simulink model "TTS2_EXT"  (R2024b)
settings: Solver=FixedStepAuto  StartTime=0.0  StopTime=inf  FixedStep=0.01  RelTol=1e-3
model workspace (MAT data in the model file):
  amp_f1 = -100
  amp_f10 = 0.5
  amp_f11 = -0.1
  amp_f12 = 1
  amp_f13 = 0.5
  amp_f14 = -20
  amp_f15 = 0.5
  amp_f16 = 0.5
  amp_f17 = 20
  amp_f18 = -30
  amp_f19 = 0.1
  amp_f2 = -20
  amp_f20 = -20
  amp_f21 = 20
  amp_f3 = -30
  amp_f4 = -30
  amp_f5 = -10
  amp_f51 = -10
  amp_f52 = -30
  amp_f53 = -30
  amp_f54 = 20
  amp_f55 = -100
  amp_f6 = -30
  amp_f7 = -30
  amp_f8 = -30
  amp_f9 = 1
  from_f1 = 570
  from_f10 = 5970
  from_f11 = 6570
  from_f12 = 7170
  from_f13 = 7770
  from_f14 = 8370
  from_f15 = 8970
  from_f16 = 9570
  from_f17 = 10170
  from_f18 = 10770
  from_f19 = 11370
  from_f2 = 1170
  from_f20 = 11970
  from_f21 = 12570
  from_f3 = 1770
  from_f4 = 2370
  from_f5 = 2970
  from_f51 = 13170
  from_f52 = 13770
  from_f53 = 14370
  from_f54 = 14970
  from_f55 = 15570
  from_f6 = 3570
  from_f7 = 4170
  from_f8 = 4770
  from_f9 = 5370
libraries: simulink x52, lab310_library x26, opclib x3
(part 1 of 3)
settings Model: Creator=tanas  LastModifiedBy=pchoi
settings DataIOCC: ReturnWorkspaceOutputs=off
settings OptimizationCC: ReuseModelBlockBuffer=off
settings DebuggingCC: UnconnectedInputMsg=warning  UnconnectedOutputMsg=warning  UnconnectedLineMsg=warning  ArithmeticOperatorsInVariantConditions=warning
settings ModelReferenceCC: EnableRefExpFcnMdlSchedulingChecks=on
settings SFSimCC: CustomCodeUndefinedFunction=UseInterfaceOnly
settings RTWCC: GPUComputeCapability=3.5

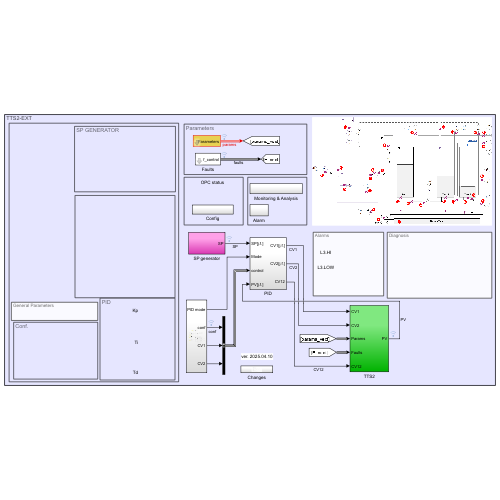
[thumbnail: Simulink's stored preview of the top-level diagram]
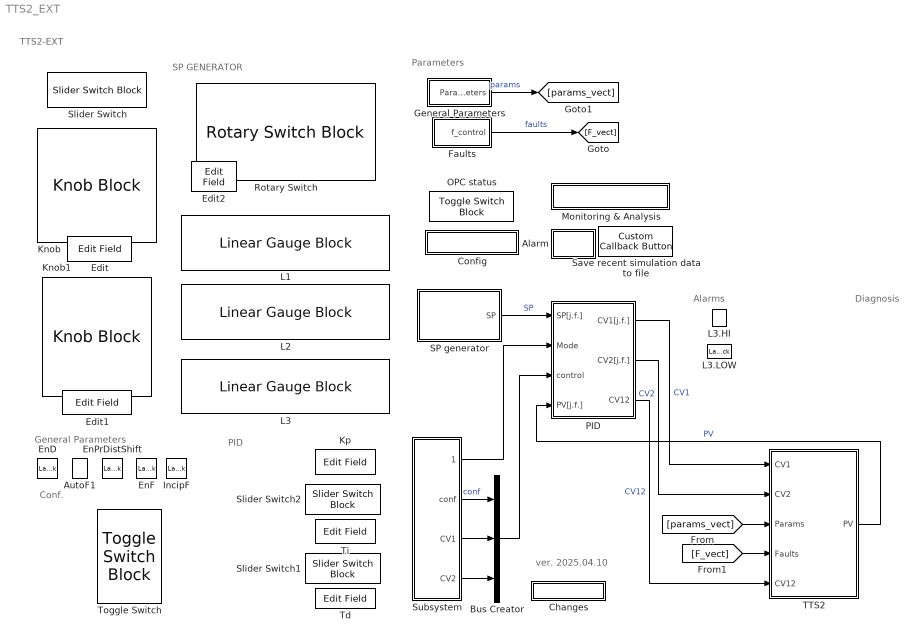
== system TTS2_EXT ==
  note: ver. 2025.04.10
  note: General Parameters
  note: Parameters
  note: PID
  note: Conf.
  note: TTS2-EXT
  note: SP GENERATOR
  note: Alarms
  note: Diagnosis
  Alarm : Subsystem
  AutoF1 : LampBlock
  Bus Creator : BusCreator  Inputs=3
  Changes : Subsystem
  Config : Subsystem
  Edit : EditField  LabelPosition=Hide  ShowInitialText=on  Alignment=Center
  Edit1 : EditField  LabelPosition=Hide  ShowInitialText=on  Alignment=Center
  Edit2 : EditField  LabelPosition=Hide  ShowInitialText=on  Alignment=Center
  EnD : LampBlock
  EnF : LampBlock
  EnPrDistShift : LampBlock
  Faults : Subsystem  mask{EnF=on, IncipF=off, st=300, w_f1=praca, p_f1=on, t_f1=0, w_f2=0, p_f2=on, t_f2=0, w_f3=0, p_f3=on, t_f3=0, w_f4=0, p_f4=on, t_f4=0, w_f5=0, p_f5=on, t_f5=0, w_f6=0, p_f6=on, t_f6=0, w_f7=0, p_f7=on, t_f7=0, w_f8=0, p_f8=on, t_f8=0, w_f9=0, p_f9=on, t_f9=0, w_f10=0, p_f10=on, t_f10=0, w_f11=0, p_f11=on, t_f11=100, w_f12=0, p_f12=on, t_f12=0, w_f13=0, p_f13=on, t_f13=0, w_f14=0, p_f14=on, t_f14=0, w_f15=0, p_f15=on, t_f15=0, w_f16=0, p_f16=on, t_f16=0, w_f17=0, p_f17=on, t_f17=0, w_f18=0, p_f18=on, t_f18=0, w_f19=0, p_f19=on, t_f19=0, w_f20=0, p_f20=on, t_f20=0, w_f21=0, p_f21=on, t_f21=0, w_f51=0, p_f51=on, t_f51=0, w_f52=0, p_f52=on, t_f52=0, w_f53=0, p_f53=on, t_f53=0, w_f54=0, p_f54=on, t_f54=0, w_f55=brak, p_f55=on, t_f55=0}
      mask prompts: EnF "Enable faults"; IncipF "Tryb uszkodzeń narastających"; st "Czas narastania"; w_f1 "Wartość"; p_f1 "Czy symulacja uszkodzenia włączona?"; t_f1 "Czas startu"; w_f2 "Wartość [-100,0]"; p_f2 "Czy symulacja uszkodzenia włączona?"; t_f2 "Czas startu"; w_f3 "Wartość [-100,100]"; p_f3 "Czy symulacja uszkodzenia włączona?"; t_f3 "Czas startu"; w_f4 "Wartość [-100,0]"; p_f4 "Czy symulacja uszkodzenia włączona?"; t_f4 "Czas startu"; w_f5 "Wartość [-100,100]"; p_f5 "Czy symulacja uszkodzenia włączona?"; t_f5 "Czas startu"; w_f6 "Wartość [-100,100]"; p_f6 "Czy symulacja uszkodzenia włączona?"; t_f6 "Czas startu"; w_f7 "Wartość [-100,100]"; p_f7 "Czy symulacja uszkodzenia włączona?"; t_f7 "Czas startu"; w_f8 "Wartość [-100,100]"; p_f8 "Czy symulacja uszkodzenia włączona?"; t_f8 "Czas startu"; w_f9 "Wartość [0,1]"; p_f9 "Czy symulacja uszkodzenia włączona?"; t_f9 "Czas startu"; w_f10 "Wartość [0,1]"; p_f10 "Czy symulacja uszkodzenia włączona?"; t_f10 "Czas startu"; w_f11 "Wartość [-1,1]"; p_f11 "Czy symulacja uszkodzenia włączona?"; t_f11 "Czas startu"; w_f12 "Wartość [0,1]"; p_f12 "Czy symulacja uszkodzenia włączona?"; t_f12 "Czas startu"; w_f13 "Wartość [0,1]"; p_f13 "Czy symulacja uszkodzenia włączona?"; t_f13 "Czas startu"; w_f14 "Wartość [-100,100]"; p_f14 "Czy symulacja uszkodzenia włączona?"; t_f14 "Czas startu"; w_f15 "Wartość [0,1]"; p_f15 "Czy symulacja uszkodzenia włączona?"; t_f15 "Czas startu"; w_f16 "Wartość [0,1]"; p_f16 "Czy symulacja uszkodzenia włączona?"; t_f16 "Czas startu"; w_f17 "Wartość [-100,100]"; p_f17 "Czy symulacja uszkodzenia włączona?"; t_f17 "Czas startu"; w_f18 "Wartość [-100,100]"; p_f18 "Czy symulacja uszkodzenia włączona?"; t_f18 "Czas startu"; w_f19 "Wartość [-1,1]"; p_f19 "Czy symulacja uszkodzenia włączona?"; t_f19 "Czas startu"; w_f20 "Wartość [-100,100]"; p_f20 "Czy symulacja uszkodzenia włączona?"; t_f20 "Czas startu"; w_f21 "Wartość [-100,100]"; p_f21 "Czy symulacja uszkodzenia włączona?"; t_f21 "Czas startu"; w_f51 "Wartość [-100,100]"; p_f51 "Czy symulacja uszkodzenia włączona?"; t_f51 "Czas startu"; w_f52 "Wartość [-100,100]"; p_f52 "Czy symulacja uszkodzenia włączona?"; t_f52 "Czas startu"; w_f53 "Wartość [-100,100]"; p_f53 "Czy symulacja uszkodzenia włączona?"; t_f53 "Czas startu"; w_f54 "Wartość [-100,100]"; p_f54 "Czy symulacja uszkodzenia włączona?"; t_f54 "Czas startu"; w_f55 "Wartość"; p_f55 "Czy symulacja uszkodzenia włączona?"; t_f55 "Czas startu"
      mask DialogControl Container70 Prompt: Incipient faults
      mask DialogControl Container4 Prompt: f1-Zatrzymanie pracy pompy
      mask DialogControl Container4_copy Prompt: f2-Spadek wydajności pompy
      mask DialogControl Container6 Prompt: f3-Uszkodzenie w torze sygnału sterującego CV
      mask DialogControl Container8 Prompt: f4-Uszkodzenie siłownika zaworu regulacyjnego
      mask DialogControl Container10 Prompt: f5-Uszkodzenie toru pomiarowego położenia zaworu G1
      mask DialogControl Container12 Prompt: f6-Uszkodzenie grzyba lub gniazda zaworu regulacyjnego V1
      mask DialogControl Container14 Prompt: f7-Uszkodzenie toru pomiarowego przepływu F1
      mask DialogControl Container16 Prompt: f8-Uszkodzenie toru pomiarowego poziomu L11
      mask DialogControl Container18 Prompt: f9-Przeciek ze zbiornika 1
      mask DialogControl Container20 Prompt: f10-Częściowe przytkanie kanału pomiędzy zbiornikami 1 i 2
      mask DialogControl Container22 Prompt: f11-Uszkodzenie toru pomiarowego poziomu L21
      mask DialogControl Container41 Prompt: f12-Przeciek ze zbiornika 2
      mask DialogControl Container42 Prompt: f13-Częściowe przytkanie kanału pomiędzy zbiornikami 2 i 3
      mask DialogControl Container44 Prompt: f14-Uszkodzenie toru pomiarowego poziomu L31
      mask DialogControl Container46 Prompt: f15-Przeciek ze zbiornika 3
      mask DialogControl Container48 Prompt: f16-Częściowe przytkanie odpływu
      mask DialogControl Container50 Prompt: f17-Uszkodzenie toru pomiarowego przepływu F2
      mask DialogControl Container52 Prompt: f18-Uszkodzenie toru pomiarowego poziomu L12
      mask DialogControl Container54 Prompt: f19-Uszkodzenie toru pomiarowego poziomu L22
      mask DialogControl Container56 Prompt: f20-Uszkodzenie toru pomiarowego poziomu L32
      mask DialogControl Container58 Prompt: f21-Uszkodzenie toru pomiarowego ciśnienia P
      mask DialogControl Container60 Prompt: f51-Uszkodzenie toru pomiarowego położenia zaworu G2
      mask DialogControl Container62 Prompt: f52-Uszkodzenie przetwornika różnicy ciśnienia dP
      mask DialogControl Container64 Prompt: f53-Uszkodzenie grzyba lub gniazda zaworu regulacyjnego V2
      mask DialogControl Container66 Prompt: f54-Uszkodzenie toru pomiarowego przepływu F3
      mask DialogControl Container68 Prompt: f55-Nieoczekiwane otwarcie / zamknięcie kanału miedzy zbiornikami 1 i 2
  "General Parameters " : Subsystem  mask(General Parameters){EnD=on, PrDistValue=20, EnPrDist=off, PrDistShift=80, EnPrDistShift=on}
      mask prompts: EnD "Zakłócenia pomiarowe (EnD)"; PrDistValue "wartość fluktuacji [%]"; EnPrDist "włączenie fluktuacji (EnPrDist)"; PrDistShift "wartość stala [%]"; EnPrDistShift "włączenie wartości stałej (EnPrDistShift)"
      mask DialogControl Control2 Prompt: włączanie / wyłącznie zakłóceń pomiarowych (praktycznie zawsze włączone) (wył - do wykorzystania przy badaniu sterowania)
      mask DialogControl Container16 Prompt: Zakłócenia procesowe
      mask DialogControl Control3 Prompt: włączanie / wyłącznie zmian - plus/minu [%] sygnału sterującego pompy zakłócenia
      mask DialogControl Control7 Prompt: włączanie / wyłącznie stałej wartości - [%] sygnału sterującego pompy zakłócenia
  IncipF : LampBlock
  Knob : KnobBlock  TickInterval=5
  Knob1 : KnobBlock  TickInterval=5
  Kp : EditField  LabelPosition=Hide  ShowInitialText=on  Alignment=Center
  L1 : LinearGaugeBlock  ScaleMax=1
  L2 : LinearGaugeBlock  ScaleMax=1
  L3 : LinearGaugeBlock  ScaleMax=1
  L3.HI : LampBlock  LabelPosition=Hide
  L3.LOW : LampBlock  LabelPosition=Hide
  Monitoring & Analysis : Subsystem
  OPC status : ToggleSwitchBlock  LabelPosition=Hide
      settings: Values={{'Off', 'On'}, [0 1]}
  PID : Subsystem
  Rotary Switch : RotarySwitchBlock
      settings: Values={{'SP Manual', 'Sine Signal', 'Lookup table'}, [1 2 3]}
  SP generator : Subsystem
  Save recent simulation data to file : CustomCallbackButton  Configuration="{\"components\":[{\"name\":\"BackgroundImageComponent\",\"settings\":{\"image\":{\"size\":[0,0],\"src\":\"default\",\"srcOrientation\":\"Right\"},\"position\":[0,0,1,1]}},{\"name\":\"ButtonStateComponent\",\"settings\":{\"buttonType\":\"momentary\",\"clickFcn\":\"exist tout var; \\nt_e=ans;\\nexist simout var; \\ns_e=ans;\\nif (t_e==1 && s_e==1)\\n    \\n    t=datetime;\\n    DateString=join(string(int16(datevec(t))),\\\"_\\\");\\n    filename =join(['TTS2_ext_symulationdata',DateString,'.xlsx'],\\\"_\\\");\\n    Time=tout;\\n\\n    SP=simout(:,1);\\n    CV= simout(:,2);\\n    PV= simout(:,3);\\n    G1= simout(:,4);\\n    F1= simout(:,5);\\n    L11= simout(:,6);\\n    L12= simout(:,7);\\n    L21= simout(:,8);\\n    L22= simout(:,9);\\n    L31= simout(:,10);\\n    L32= simout(:,11);\\n    F2= simout(:,12);\\n    P1= simout(:,13);\\n    G2= simout(:,14);\\n    dP= simout(:,15);\\n    F3= simout(:,16);\\n    G3= simout(:,17);\\n    CV1= simout(:,18);\\n    CV2= simout(:,19);\\n    conf= simout(:,20);\\n\\n    T=table(Time,SP,CV,G1,F1,L11,L12,L21,L22,L31,L32,F2,P1,G2,dP,F3,G3,CV1,CV2);\\n    writetable(T,filename);\\nelse\\n    disp(\\\"Brak danych do zapisu\\\")\\nend\\n\\nclear(\\\"t_e\\\", \\\"s_e\\\");\",\"onValue\":1,\"position\":[0,0,1,1],\"pressDelay\":\"500\",\"pressFcn\":\"\",\"repeatInterval\":\"0\",\"states\":[{\"horizontalAlignment\":\"center\",\"image\":{\"position\":[0,0,1,1],\"size\":[1,1],\"src\":\"default\",\"srcOrientation\":\"Right\"},\"label\":{\"color\":[0.01176470588,0.01176470588,0.01176470588,1],\"icon\":{\"size\":[0,0],\"src\":\"default\",\"srcOrientation\":\"Right\"},\"iconPlacement\":\"left\",\"opacity\":1,\"show\":true,\"text\":{\"content\":\"Save to file\",\"font\":\"Helvetica\"}},\"labelOffset\":[0,0],\"verticalAlignment\":\"middle\"},{\"horizontalAlignment\":\"center\",\"image\":{\"position\":[0,0,1,1],\"size\":[1,1],\"src\":\"default\",\"srcOrientation\":\"Right\"},\"label\":{\"color\":[0.01176470588,0.01176470588,0.01176470588,1],\"icon\":{\"size\":[0,0],\"src\":\"default\",\"srcOrientation\":\"Right\"},\"iconPlacement\":\"left\",\"opacity\":1,\"show\":true,\"text\":{\"content\":\"Save to file\",\"font\":\"Helvetica\"}},\"labelOffset\":[0,0],\"verticalAlignment\":\"middle\"},{\"horizontalAlignment\":\"center\",\"image\":{\"position\":[0,0,1,1],\"size\":[1,1],\"src\":\"default\",\"srcOrientation\":\"Right\"},\"label\":{\"color\":[0.01176470588,0.01176470588,0.01176470588,1],\"icon\":{\"size\":[0,0],\"src\":\"default\",\"srcOrientation\":\"Right\"},\"iconPlacement\":\"left\",\"opacity\":1,\"show\":true,\"text\":{\"content\":\"Save to file\",\"font\":\"Helvetica\"}},\"labelOffset\":[0,0],\"verticalAlignment\":\"middle\"},{\"horizontalAlignment\":\"center\",\"image\":{\"position\":[0,0,1,1],\"size\":[1,1],\"src\":\"default\",\"srcOrientation\":\"Right\"},\"label\":{\"color\":[0.01176470588,0.01176470588,0.01176470588,1],\"icon\":{\"size\":[0,0],\"src\":\"default\",\"srcOrientation\":\"Right\"},\"iconPlacement\":\"left\",\"opacity\":1,\"show\":true,\"text\":{\"content\":\"Save to file\",\"font\":\"Helvetica\"}},\"labelOffset\":[0,0],\"verticalAlignment\":\"middle\"}]}},{\"name\":\"ForegroundImageComponent\",\"settings\":{\"image\":{\"size\":[0,0],\"src\":\"default\",\"srcOrientation\":\"Right\"},\"isForeground\":1,\"position\":[0,0,1,1]}}],\"settings\":{\"BindingType\":\"standalone\",\"backgroundColor\":[244,244,244,1],\"backgroundOffset\":0.2,\"backgroundOpacity\":1,\"fixedAspectRatio\":\"off\",\"foregroundColor\":[0.01176470588,0.01176470588,0.01176470588,1],\"migratedFromLegacy\":true,\"useBackgroundColor\":true,\"variant\":\"callback\",\"version\":\"R2024b\"},\"type\":\"Button\"}"  CustomBackgroundColor="{\"color\":[0.9568627450980393,0.9568627450980393,0.9568627450980393],\"show\":true}"
  Slider Switch : SliderSwitchBlock
      settings: Values={{'Auto', 'Manual'}, [1 2]}
  Slider Switch1 : SliderSwitchBlock
      settings: Values={{'Off', 'On'}, [0 1]}
  Slider Switch2 : SliderSwitchBlock
      settings: Values={{'Off', 'On'}, [0 1]}
  Subsystem : Subsystem
  TTS2 : Subsystem
  Td : EditField  LabelPosition=Hide  ShowInitialText=on  Alignment=Center
  Ti : EditField  LabelPosition=Hide  ShowInitialText=on  Alignment=Center
  Toggle Switch : ToggleSwitchBlock
      settings: Values={{'Valve V1', 'Valve V2'}, [1 2]}
  wires:
  Faults/1(f_control) -> [F_vect]  "faults"
  "General Parameters "/1(Parameters) -> [params_vect]  "params"
  Subsystem/4(CV2) -> Bus Creator/3
  [params_vect] -> TTS2/3(Params)
  [F_vect] -> TTS2/4(Faults)
  PID/1(CV1[j.f.]) -> TTS2/1(CV1)  "CV1"
  SP generator/1(SP) -> PID/1(SP[j.f.])  "SP"
  Subsystem/1(PID mode) -> PID/2(Mode)
  Subsystem/3(CV1) -> Bus Creator/2
  Bus Creator/1 -> PID/3(control)
  TTS2/1(PV) -> PID/4(PV[j.f.])  "PV"
  Subsystem/2(conf) -> Bus Creator/1  "conf"
  PID/2(CV2[j.f.]) -> TTS2/2(CV2)  "CV2"
  PID/3(CV12) -> TTS2/5(CV12)  "CV12"

== system TTS2_EXT/Alarm ==
  Compare To Constant : simulink/Logic and Bit Operations/Compare To Constant  relop=<=  const=0.059  OutDataTypeStr=boolean
  Compare To Constant1 : simulink/Logic and Bit Operations/Compare To Constant  relop=<=  const=0.055  OutDataTypeStr=boolean
  Compare To Constant2 : simulink/Logic and Bit Operations/Compare To Constant  relop=>=  const=0.0635  OutDataTypeStr=boolean
  Compare To Constant3 : simulink/Logic and Bit Operations/Compare To Constant  relop=>=  const=0.064  OutDataTypeStr=boolean
  Sum : Sum  Inputs=|+|+|
  Sum1 : Sum  Inputs=|+|+|
  Terminator : Terminator
  Terminator1 : Terminator
  wires:
  [PV] -> Compare To Constant/1, Compare To Constant1/1, Compare To Constant3/1, Compare To Constant2/1
  Sum/1 -> Terminator/1  "L3.LOW"
  Compare To Constant/1 -> Sum/1
  Compare To Constant1/1 -> Sum/2
  Compare To Constant2/1 -> Sum1/1
  Compare To Constant3/1 -> Sum1/2
  Sum1/1 -> Terminator1/1  "L3.HI"

== system TTS2_EXT/Changes ==
  note: Dziennik zmian:
      | 2023-05-11 : konfiguracja OPC dla konfiguracji podstawowej
      | 2023-05-25 : pełna konfiguracja OPC
      | 2023-11-26: a) zmiana konfiguracji jednym sygnałem (przełączenie sterownika V1->V2 i zmiana stanu zaworu V12)
      | b) podłączenie wszystkich sygnałów do bloku analizy
      | c) różni SEED dla zakłóceń
      | d) ujednolicenie nazw wewnętrznych z dokumentacją
      | e) uporządkowanie sygnałów w Data Inspector
      | f) dodanie sterowania wielkością zakłóceń procesowych
      | g) usprawienie symulacji uszkodzeń w zakresie:
      | - Uszkodzenie (wielkość, symulowane od) - parametry bloku "Faults"
      | - Powolinarastające - uruchamia płynne przejście do ustawionej wartości uszkodzenia w usalonym czasie (parametr stały)
      | - AutF - odtwarza automatyczne uszkodzenia w założonym czasie i o założonej wartości (parametry stałe)
      | 2024-01-16 : wprowadzenie antiwindup dla trybu pracy ręcznej regulatora
      | 2024-04-30: a) Wprowadzenie fizycznego ograniczenia <0,1> na ustawienie grzyba zaworu
      | b) Wprowadzenie fizycznego ograniczenia <0, max> na zmianę powierzchni czynnej zaworu
      | 2024-11-13: a) Zmiana sterowania uszkodzeniami (zmiana incipient, przeniesienie parametrów z grupy ogólnych)
      | b) Poprawa uszkodzenia f55
      | c) Zmiany sterowania zaworami V1 i V3 w funkcji konfiguracji obiektu
      | d) Wprowadzenie bliblioteki lab310_library
      | e) Poprawa obsługi sygnału konfiguracji z OPC
      | 2024-11-19: a) Wprowadzenie jawnej konwersji bool->double
      | 2024-12-01: a) Poprawa wyliczania spadku ciśnienia zasilania przy pracy V2
      | 2025-04-10: a) Zamiana nazw F2 z F3, G3 na G12
      | b) Zmiana zakresu sygnałów SP_mode, PID_mode, OPER_mode

== system TTS2_EXT/Config ==
  Bus Selector : BusSelector  OutputSignals=P1,G1,F1,G2,dP2,F2,G12,L11,L12,L21,L22,L31,L32,F3
  Demux : Demux  Outputs=6
  Mux : Mux  Inputs=19
  OPCstatus : Constant  OutMin=0  OutMax=1
  Subsystem : Subsystem
  Subsystem1 : Subsystem
  tag scope: CVG1man=global, CVG2man=global, OPCstatus=global, OPERmode=global, PIDmode=global, SPman=global, SPmode=global
  wires:
  [SP] -> Mux/1
  [CV] -> Mux/2
  OPCstatus/1 -> [OPCstatus], Subsystem/Enable, Subsystem1/Enable  "OPCstatus"
  [data] -> Bus Selector/1
  Bus Selector/1 -> Mux/3  "<P1>"
  [CVG1] -> Mux/4
  Bus Selector/2 -> Mux/5  "<G1>"
  Bus Selector/3 -> Mux/6  "<F1>"
  [CVG2] -> Mux/7
  Bus Selector/4 -> Mux/8  "<G2>"
  Bus Selector/5 -> Mux/9  "<dP2>"
  Bus Selector/6 -> Mux/10  "<F2>"
  [CVG12] -> Mux/11
  Bus Selector/7 -> Mux/12  "<G12>"
  Bus Selector/8 -> Mux/13  "<L11>"
  Bus Selector/9 -> Mux/14  "<L12>"
  Bus Selector/10 -> Mux/15  "<L21>"
  Bus Selector/11 -> Mux/16  "<L22>"
  Bus Selector/12 -> Mux/17  "<L31>"
  Bus Selector/13 -> Mux/18  "<L32>"
  Bus Selector/14 -> Mux/19  "<F3>"
  Mux/1 -> Subsystem/1(In1)
  Subsystem1/1(Out1) -> Demux/1
  Demux/1 -> [OPERmode]
  Demux/2 -> [PIDmode]
  Demux/3 -> [SPmode]
  Demux/4 -> [SPman]
  Demux/5 -> [CVG1man]
  Demux/6 -> [CVG2man]

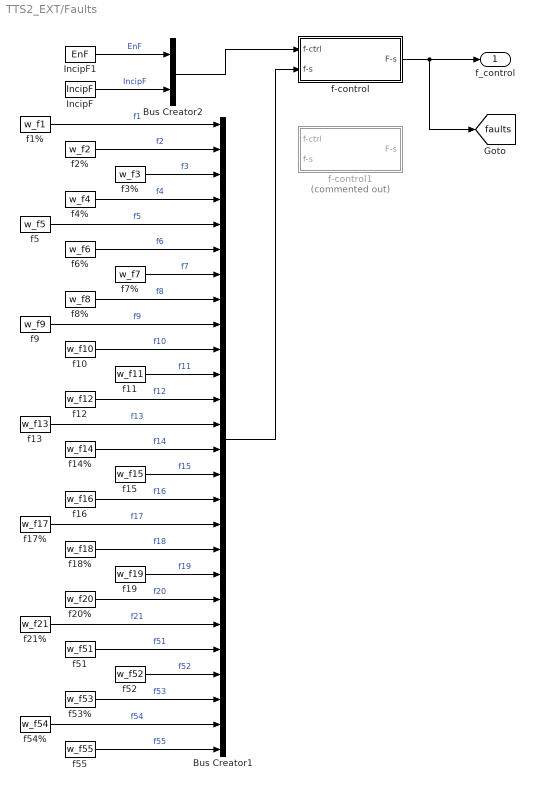
== system TTS2_EXT/Faults ==
  Bus Creator1 : BusCreator  Inputs=26
  Bus Creator2 : BusCreator  Inputs=2
  IncipF : Constant  Value=IncipF  OutMin=0  OutMax=1
  IncipF1 : Constant  Value=EnF  OutMin=0  OutMax=1
  f-control : Subsystem
  f-control1 : Subsystem  Commented=on
  f1% : Constant  Value=w_f1  OutMin=-100  OutMax=0
  f10 : Constant  Value=w_f10  OutMin=0  OutMax=1
  f11 : Constant  Value=w_f11  OutMin=-1  OutMax=1
  f12 : Constant  Value=w_f12  OutMin=0  OutMax=1
  f13 : Constant  Value=w_f13  OutMin=0  OutMax=1
  f14% : Constant  Value=w_f14  OutMin=-100  OutMax=100
  f15 : Constant  Value=w_f15  OutMin=0  OutMax=1
  f16 : Constant  Value=w_f16  OutMin=0  OutMax=1
  f17% : Constant  Value=w_f17  OutMin=-100  OutMax=100
  f18% : Constant  Value=w_f18  OutMin=-100  OutMax=100
  f19 : Constant  Value=w_f19  OutMin=-1  OutMax=1
  f2% : Constant  Value=w_f2  OutMin=-100  OutMax=0
  f20% : Constant  Value=w_f20  OutMin=-100  OutMax=100
  f21% : Constant  Value=w_f21  OutMin=-100  OutMax=100
  f3% : Constant  Value=w_f3  OutMin=-100  OutMax=100
  f4% : Constant  Value=w_f4  OutMin=-100  OutMax=0
  f5 : Constant  Value=w_f5  OutMin=-100  OutMax=100
  f51 : Constant  Value=w_f51  OutMin=-100  OutMax=100
  f52 : Constant  Value=w_f52  OutMin=-100  OutMax=100
  f53% : Constant  Value=w_f53  OutMin=-100  OutMax=100
  f54% : Constant  Value=w_f54  OutMin=-100  OutMax=100
  f55 : Constant  Value=w_f55  OutMin=0  OutMax=1
  f6% : Constant  Value=w_f6  OutMin=-100  OutMax=100
  f7% : Constant  Value=w_f7  OutMin=-100  OutMax=100
  f8% : Constant  Value=w_f8  OutMin=-100  OutMax=100
  f9 : Constant  Value=w_f9  OutMin=0  OutMax=1
  f_control : Outport  VectorParamsAs1DForOutWhenUnconnected=off
  tag scope: faults=global
  wires:
  f1%/1 -> Bus Creator1/1  "f1"
  f14%/1 -> Bus Creator1/14  "f14"
  f5/1 -> Bus Creator1/5  "f5"
  f9/1 -> Bus Creator1/9  "f9"
  Bus Creator1/1 -> f-control/2(f-s)
  f3%/1 -> Bus Creator1/3  "f3"
  f10/1 -> Bus Creator1/10  "f10"
  f12/1 -> Bus Creator1/12  "f12"
  f4%/1 -> Bus Creator1/4  "f4"
  f2%/1 -> Bus Creator1/2  "f2"
  f11/1 -> Bus Creator1/11  "f11"
  f15/1 -> Bus Creator1/15  "f15"
  f6%/1 -> Bus Creator1/6  "f6"
  f7%/1 -> Bus Creator1/7  "f7"
  f8%/1 -> Bus Creator1/8  "f8"
  f13/1 -> Bus Creator1/13  "f13"
  f-control/1(F-s) -> [faults], f_control/1
  f16/1 -> Bus Creator1/16  "f16"
  f17%/1 -> Bus Creator1/17  "f17"
  f18%/1 -> Bus Creator1/18  "f18"
  f19/1 -> Bus Creator1/19  "f19"
  f20%/1 -> Bus Creator1/20  "f20"
  f21%/1 -> Bus Creator1/21  "f21"
  f51/1 -> Bus Creator1/22  "f51"
  f52/1 -> Bus Creator1/23  "f52"
  f53%/1 -> Bus Creator1/24  "f53"
  f54%/1 -> Bus Creator1/25  "f54"
  f55/1 -> Bus Creator1/26  "f55"
  IncipF/1 -> Bus Creator2/2  "IncipF"
  Bus Creator2/1 -> f-control/1(f-ctrl)
  IncipF1/1 -> Bus Creator2/1  "EnF"

== system TTS2_EXT/General Parameters  ==
  Bus Creator : BusCreator  Inputs=5
  EnD : Constant  Value=EnD  OutMin=0  OutMax=1
  EnPrDist : Constant  Value=EnPrDist  OutMin=0  OutMax=1
  EnPrDistShift : Constant  Value=EnPrDistShift  OutMin=0  OutMax=1
  PrDistShift : Constant  Value=PrDistShift  OutMin=0  OutMax=100
  PrDistValue : Constant  Value=PrDistValue  OutMin=0  OutMax=50
  Parameters : Outport  VectorParamsAs1DForOutWhenUnconnected=off
  wires:
  EnPrDistShift/1 -> Bus Creator/3  "EnPrDistShift"
  EnD/1 -> Bus Creator/1  "EnD"
  EnPrDist/1 -> Bus Creator/2  "EnPrDist"
  Bus Creator/1 -> Parameters/1
  PrDistValue/1 -> Bus Creator/4  "PrDistValue"
  PrDistShift/1 -> Bus Creator/5  "PrDistShift"

== system TTS2_EXT/Monitoring & Analysis ==
  Export data : Subsystem
  Scopes : Subsystem
  Terminator : Terminator
  Terminator1 : Terminator
  wires:
  [SP] -> Scopes/2(SP), Export data/1(SP)
  [CV] -> Export data/2(CV), Scopes/3(CV)
  [e] -> Scopes/1(e)
  [data] -> Scopes/4(data), Export data/4(data)
  [PV] -> Export data/3(PV)
  [faults] -> Terminator/1
  [dist] -> Terminator1/1
  [CVG1] -> Export data/5(CVG1)
  [CVG2] -> Export data/6(CVG2)
  [conf] -> Export data/7(conf)

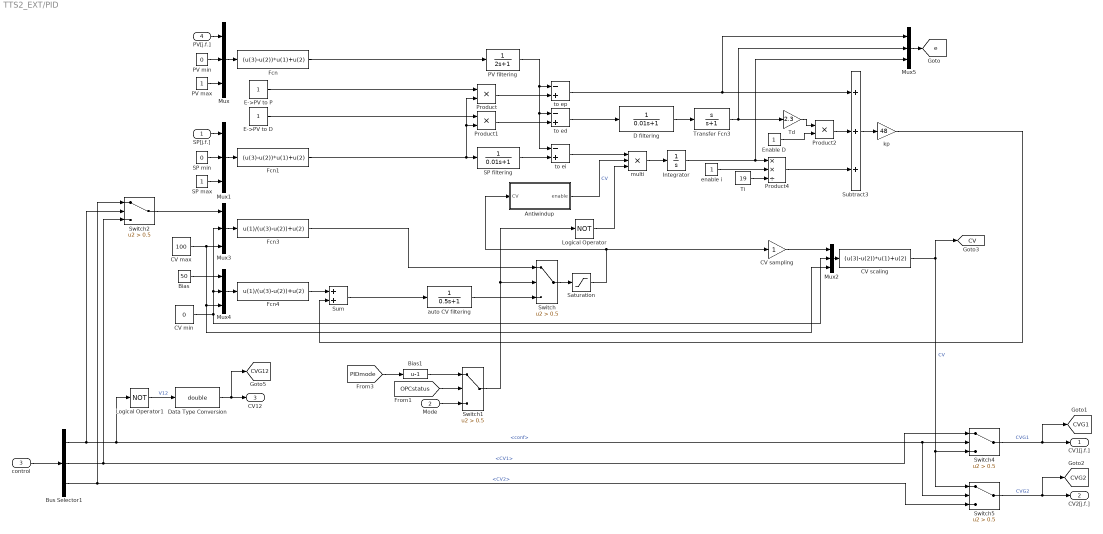
== system TTS2_EXT/PID ==
  SP[j.f.] : Inport
  Mode : Inport  Port=2
  control : Inport  Port=3
  PV[j.f.] : Inport  Port=4
  Antiwindup : Subsystem
  Bias : Constant  Value=50
  Bias1 : Bias  Bias=-1  SaturateOnIntegerOverflow=off
  Bus Selector1 : BusSelector  OutputSignals=conf,CV1,CV2
  CV max : Constant  Value=100
  CV min : Constant  Value=0
  CV sampling : Gain
  CV scaling : Fcn  Expr=(u(3)-u(2))*u(1)+u(2)
  D filtering : TransferFcn  Denominator=[0.01 1]
  Data Type Conversion : DataTypeConversion  OutDataTypeStr=double  SaturateOnIntegerOverflow=off  RndMeth=Floor
  E->PV to D : Constant
  E->PV to P : Constant
  Enable D : Constant
  Fcn : Fcn  Expr=(u(3)-u(2))*u(1)+u(2)
  Fcn1 : Fcn  Expr=(u(3)-u(2))*u(1)+u(2)
  Fcn3 : Fcn  Expr=u(1)/(u(3)-u(2))+u(2)
  Fcn4 : Fcn  Expr=u(1)/(u(3)-u(2))+u(2)
  Integrator : Integrator
  Logical Operator : Logic  Operator=NOT  AllPortsSameDT=off  OutDataTypeStr=boolean
  Logical Operator1 : Logic  Operator=NOT  AllPortsSameDT=off  OutDataTypeStr=boolean
  Mux{,1..5} (6 alike) : Mux  Inputs=3
  PV filtering : TransferFcn  Denominator=[2 1]
  PV max : Constant
  PV min : Constant  Value=0
  Product : Product
  Product1 : Product
  Product2 : Product
  Product4 : Product  Inputs=**/
  SP filtering : TransferFcn  Denominator=[0.01 1]
  SP max : Constant
  SP min : Constant  Value=0
  Saturation : Saturate  UpperLimit=1  LowerLimit=0
  Subtract3 : Sum  Inputs=+++
  Sum : Sum
  Switch{,1..2,4..5} (5 alike) : Switch  Criteria=u2 > Threshold  Threshold=0.5  SaturateOnIntegerOverflow=off  InputSameDT=off
  Td : Gain  Gain=2.3
  Ti : Constant  Value=19
  Transfer Fcn3 : TransferFcn  Numerator=[1 0]  Denominator=[1 1]
  auto CV filtering : TransferFcn  Denominator=[0.5 1]
  enable i : Constant
  kp : Gain  Gain=48
  multi : Product  Inputs=3
  to ed : Sum  Inputs=-+
  to ei : Sum  Inputs=-+  OutMin=[0]  OutMax=[0]
  to ep : Sum  Inputs=-+
  CV1[j.f.] : Outport  VectorParamsAs1DForOutWhenUnconnected=off
  CV2[j.f.] : Outport  Port=2  VectorParamsAs1DForOutWhenUnconnected=off
  CV12 : Outport  Port=3
  tag scope: CV=global, CVG12=global, CVG1=global, CVG2=global, e=global
  wires:
  Mux/1 -> Fcn/1
  PV min/1 -> Mux/2
  PV max/1 -> Mux/3
  PV filtering/1 -> to ei/1, to ed/1, to ep/1
  E->PV to D/1 -> Product1/1
  E->PV to P/1 -> Product/1
  Product/1 -> to ep/2
  Product1/1 -> to ed/2
  Mux1/1 -> Fcn1/1
  SP[j.f.]/1 -> Mux1/1
  SP min/1 -> Mux1/2
  SP max/1 -> Mux1/3
  Fcn1/1 -> SP filtering/1, Product/2, Product1/2
  D filtering/1 -> Transfer Fcn3/1
  Td/1 -> Product2/1
  Enable D/1 -> Product2/2
  Product2/1 -> Subtract3/2
  to ed/1 -> D filtering/1
  to ep/1 -> Mux5/1, Subtract3/1
  Subtract3/1 -> kp/1
  multi/1 -> Integrator/1
  Integrator/1 -> Product4/1, Mux5/3
  Ti/1 -> Product4/3
  enable i/1 -> Product4/2
  Product4/1 -> Subtract3/3
  Mux2/1 -> CV scaling/1
  CV sampling/1 -> Mux2/1
  CV min/1 -> Mux2/2, Mux3/2, Mux4/2
  CV max/1 -> Mux2/3, Mux4/3, Mux3/3
  Saturation/1 -> CV sampling/1, Antiwindup/1(CV)
  Switch/1 -> Saturation/1
  Mux3/1 -> Fcn3/1
  Mux4/1 -> Fcn4/1
  Fcn4/1 -> Sum/1
  Bias/1 -> Mux4/1
  CV scaling/1 -> Switch5/1, Switch4/3, [CV]  "CV"
  Antiwindup/1(enable) -> multi/2  "CV"
  Mux5/1 -> [e]
  Transfer Fcn3/1 -> Mux5/2, Td/1
  kp/1 -> Sum/2
  to ei/1 -> multi/1
  PV[j.f.]/1 -> Mux/1
  SP filtering/1 -> to ei/2
  Fcn/1 -> PV filtering/1
  [OPCstatus] -> Switch1/2
  [PIDmode] -> Bias1/1
  Mode/1 -> Switch1/3
  Logical Operator/1 -> multi/3
  Switch1/1 -> Logical Operator/1, Switch/2
  Bias1/1 -> Switch1/1
  Sum/1 -> auto CV filtering/1
  Fcn3/1 -> Switch/1
  control/1 -> Bus Selector1/1
  Data Type Conversion/1 -> [CVG12], CV12/1
  Logical Operator1/1 -> Data Type Conversion/1  "V12"
  Switch4/1 -> [CVG1], CV1[j.f.]/1  "CVG1"
  Switch5/1 -> [CVG2], CV2[j.f.]/1  "CVG2"
  Bus Selector1/2 -> Switch2/3, Switch4/1  "<CV1>"
  Bus Selector1/3 -> Switch5/3, Switch2/1  "<CV2>"
  Bus Selector1/1 -> Switch2/2, Logical Operator1/1, Switch5/2, Switch4/2  "<conf>"
  Switch2/1 -> Mux3/1
  auto CV filtering/1 -> Switch/3

== system TTS2_EXT/SP generator ==
  1-D Lookup Table : Lookup_n-D  NumberOfTableDimensions=1  BreakpointsForDimension1=[0 300 600 900 1200 1500 1800 2100 2400 2700 3000 3300 3600 3900 4200 4500 4800 5100 5400 5700 6000 6300 6600 6900 7200 7500 7800 8100 8400 8700 9000 9300 9600 9900 10200 10500 10800 11100 11400 11700 12000 12300 12600 12900 13200 13500 13800 14100 14400 14700 15000]  Table=[0 0.65 0.14 0.22 0.08 0.35 0.45 0.6 0.41 0.5 0.75 0.2 0.47 0.25 0.7 0.93 0.34 0.8 0.53 0.7 0.28 0.61 0.22 0.68 0.83 0.5 0.9 0.29 0.12 0.45 0.2 0.86 0.7 0.04 0.48 0.28 0.83 0.5 0.39 0.83 0.6 0.87 0.67 0.36 0.3 0.93 0.33 0.71 0.31 0.15 0]  InterpMethod=Flat  InternalRulePriority=Speed  RndMeth=Simplest
  Clock : Clock
  Gain : Gain  Gain=0.42
  Multiport Switch : MultiPortSwitch  DiagnosticForDefault=Warning  SaturateOnIntegerOverflow=off  InputSameDT=off
  SP Mode : Constant  Value=2  OutMin=0  OutMax=3
  SP manual : Constant  Value=0.21  OutMin=0  OutMax=1
  Sine Wave : Sin  Amplitude=0.1  Bias=0.21  Frequency=0.006283  SampleTime=0
  Switch1 : Switch  Criteria=u2 > Threshold  SaturateOnIntegerOverflow=off  InputSameDT=off
  Switch2 : Switch  Criteria=u2 > Threshold  SaturateOnIntegerOverflow=off  InputSameDT=off
  SP : Outport  VectorParamsAs1DForOutWhenUnconnected=off
  tag scope: SP=global
  wires:
  1-D Lookup Table/1 -> Gain/1
  Sine Wave/1 -> Multiport Switch/3
  Gain/1 -> Multiport Switch/4
  Clock/1 -> 1-D Lookup Table/1
  [OPCstatus] -> Switch1/2, Switch2/2
  [SPmode] -> Switch2/1
  SP Mode/1 -> Switch2/3
  Switch2/1 -> Multiport Switch/1
  Multiport Switch/1 -> [SP], SP/1
  Switch1/1 -> Multiport Switch/2
  SP manual/1 -> Switch1/3
  [SPman] -> Switch1/1

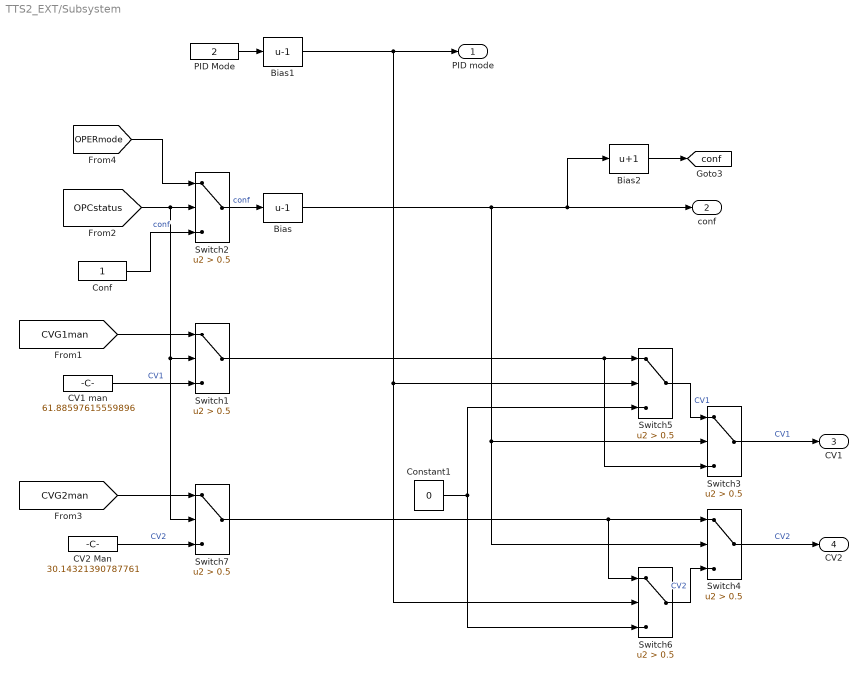
== system TTS2_EXT/Subsystem ==
  Bias : Bias  Bias=-1  SaturateOnIntegerOverflow=off
  Bias1 : Bias  Bias=-1  SaturateOnIntegerOverflow=off
  Bias2 : Bias  Bias=1  SaturateOnIntegerOverflow=off
  CV1 man : Constant  Value=61.88597615559896  OutMin=0  OutMax=100
  CV2 Man : Constant  Value=30.14321390787761  OutMin=0  OutMax=100
  Conf : Constant
  Constant1 : Constant  Value=0
  PID Mode : Constant  Value=2
  Switch{1..7} (7 alike) : Switch  Criteria=u2 > Threshold  Threshold=0.5  SaturateOnIntegerOverflow=off  InputSameDT=off
  PID mode : Outport
  conf : Outport  Port=2
  CV1 : Outport  Port=3
  CV2 : Outport  Port=4
  tag scope: conf=global
  wires:
  Conf/1 -> Switch2/3  "conf"
  [OPERmode] -> Switch2/1
  Switch2/1 -> Bias/1  "conf"
  Switch3/1 -> CV1/1  "CV1"
  Switch4/1 -> CV2/1  "CV2"
  CV1 man/1 -> Switch1/3  "CV1"
  PID Mode/1 -> Bias1/1
  Switch5/1 -> Switch3/1  "CV1"
  Switch6/1 -> Switch4/3  "CV2"
  Bias/1 -> Switch4/2, Switch3/2, conf/1, Bias2/1
  Bias1/1 -> Switch6/2, Switch5/2, PID mode/1
  Bias2/1 -> [conf]
  Constant1/1 -> Switch5/3, Switch6/3
  Switch1/1 -> Switch3/3, Switch5/1
  [CVG1man] -> Switch1/1
  [CVG2man] -> Switch7/1
  Switch7/1 -> Switch6/1, Switch4/1
  CV2 Man/1 -> Switch7/3  "CV2"
  [OPCstatus] -> Switch7/2, Switch1/2, Switch2/2

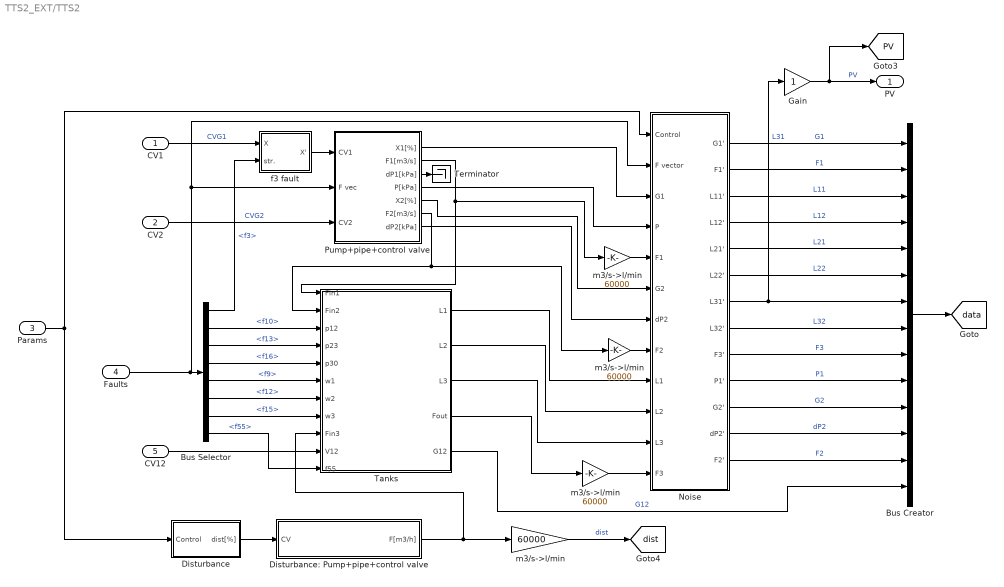
== system TTS2_EXT/TTS2 ==
  CV1 : Inport
  CV2 : Inport  Port=2
  Params : Inport  Port=3
  Faults : Inport  Port=4
  CV12 : Inport  Port=5
  Bus Creator : BusCreator  Inputs=14
  Bus Selector : BusSelector  OutputSignals=f3,f10,f13,f16,f9,f12,f15,f55
  Disturbance : Subsystem
  Disturbance: Pump+pipe+control valve : Subsystem
  Gain : Gain
  Noise : Subsystem
  Pump+pipe+control valve : Subsystem
  Tanks : Subsystem
  Terminator : Terminator
  f3 fault : Subsystem
  m3/s->l/min : Gain  Gain=60000
  "m3/s->l/min " : Gain  Gain=60000
  "m3/s->l/min  " : Gain  Gain=60000
  "m3/s->l/min   " : Gain  Gain=60000
  PV : Outport  VectorParamsAs1DForOutWhenUnconnected=off
  tag scope: PV=global, data=global, dist=global
  wires:
  Bus Creator/1 -> [data]
  Pump+pipe+control valve/7(dP2[kPa]) -> Noise/7(dP2)
  "m3/s->l/min  "/1 -> Noise/8(F2)
  Pump+pipe+control valve/6(F2[m3/s]) -> Tanks/2(Fin2), "m3/s->l/min  "/1
  Pump+pipe+control valve/5(X2[%]) -> Noise/6(G2)
  Bus Selector/8 -> Tanks/11(f55)  "<f55>"
  Disturbance: Pump+pipe+control valve/1(F[m3/h]) -> Tanks/9(Fin3), "m3/s->l/min   "/1
  Disturbance/1(dist[%]) -> Disturbance: Pump+pipe+control valve/1(CV)
  CV12/1 -> Tanks/10(V12)
  CV2/1 -> Pump+pipe+control valve/3(CV2)  "CVG2"
  CV1/1 -> f3 fault/1(X)  "CVG1"
  m3/s->l/min/1 -> Noise/5(F1)
  Pump+pipe+control valve/4(P[kPa]) -> Noise/4(P)
  Pump+pipe+control valve/2(F1[m3/s]) -> Tanks/1(Fin1), m3/s->l/min/1
  Pump+pipe+control valve/3(dP1[kPa]) -> Terminator/1
  Pump+pipe+control valve/1(X1[%]) -> Noise/3(G1)
  f3 fault/1(X') -> Pump+pipe+control valve/1(CV1)
  "m3/s->l/min "/1 -> Noise/12(F3)
  Tanks/3(L3) -> Noise/11(L3)
  Tanks/2(L2) -> Noise/10(L2)
  Tanks/1(L1) -> Noise/9(L1)
  Params/1 -> Disturbance/1(Control), Noise/1(Control)
  Bus Selector/7 -> Tanks/8(w3)  "<f15>"
  Bus Selector/6 -> Tanks/7(w2)  "<f12>"
  Bus Selector/5 -> Tanks/6(w1)  "<f9>"
  Bus Selector/4 -> Tanks/5(p30)  "<f16>"
  Bus Selector/3 -> Tanks/4(p23)  "<f13>"
  Bus Selector/2 -> Tanks/3(p12)  "<f10>"
  Bus Selector/1 -> f3 fault/2(str.)  "<f3>"
  Tanks/4(Fout) -> "m3/s->l/min "/1
  Faults/1 -> Pump+pipe+control valve/2(F vec), Noise/2(F vector), Bus Selector/1
  Tanks/5(G12) -> Bus Creator/14  "G12"
  Noise/7(L31') -> Gain/1, Bus Creator/7  "L31"
  Gain/1 -> [PV], PV/1  "PV"
  Noise/1(G1') -> Bus Creator/1  "G1"
  Noise/2(F1') -> Bus Creator/2  "F1"
  Noise/3(L11') -> Bus Creator/3  "L11"
  Noise/4(L12') -> Bus Creator/4  "L12"
  Noise/5(L21') -> Bus Creator/5  "L21"
  Noise/6(L22') -> Bus Creator/6  "L22"
  Noise/8(L32') -> Bus Creator/8  "L32"
  Noise/9(F3') -> Bus Creator/9  "F3"
  Noise/10(P1') -> Bus Creator/10  "P1"
  Noise/11(G2') -> Bus Creator/11  "G2"
  Noise/12(dP2') -> Bus Creator/12  "dP2"
  Noise/13(F2') -> Bus Creator/13  "F2"
  "m3/s->l/min   "/1 -> [dist]  "dist"

== system TTS2_EXT/Config/Subsystem ==
  In1 : Inport
  Enable : EnablePort
  OPC Configuration : opclib/OPC Configuration  opcServers=localhost/Matrikon.OPC.Simulation.1/10  errMissingItems=Error  errReadWrite=Warn  errShutdown=Error  errRTViolation=Warn  rtEnable=off  speedup=1  showLatency=off  beingUsed=on
  OPC Write : opclib/OPC Write  serverHost=localhost  serverID=Matrikon.OPC.Simulation.1  itemIDs=Bucket Brigade.SP, Bucket Brigade.CV, Bucket Brigade.P1, Bucket Brigade.CVG1, Bucket Brigade.G1, Bucket Brigade.F1, Bucket Brigade.CVG2, Bucket Brigade.G2, Bucket Brigade.dP2, Bucket Brigade.F2, Bucket Brigade.CVG12, Bucket Brigade.G12, Bucket Brigade.L11, Bucket Brigade.L12, Bucket Brigade.L21, Bucket Brigade.L22, Bucket Brigade.L31, Bucket Brigade.L32, Bucket Brigade.F3  writeMode=Synchronous  updateRate=1
  wires:
  In1/1 -> OPC Write/1

== system TTS2_EXT/Config/Subsystem1 ==
  Enable : EnablePort
  OPC Read : opclib/OPC Read  serverHost=localhost  serverID=Matrikon.OPC.Simulation.1  itemIDs=Bucket Brigade.OPERmode, Bucket Brigade.PIDmode, Bucket Brigade.SPmode, Bucket Brigade.SPman, Bucket Brigade.CVG1man, Bucket Brigade.CVG2man  readMode=Synchronous (cache)  dataType=double  updateRate=1  showQual=off  showTS=off  tsMode=Seconds since start
  Out1 : Outport
  wires:
  OPC Read/1 -> Out1/1

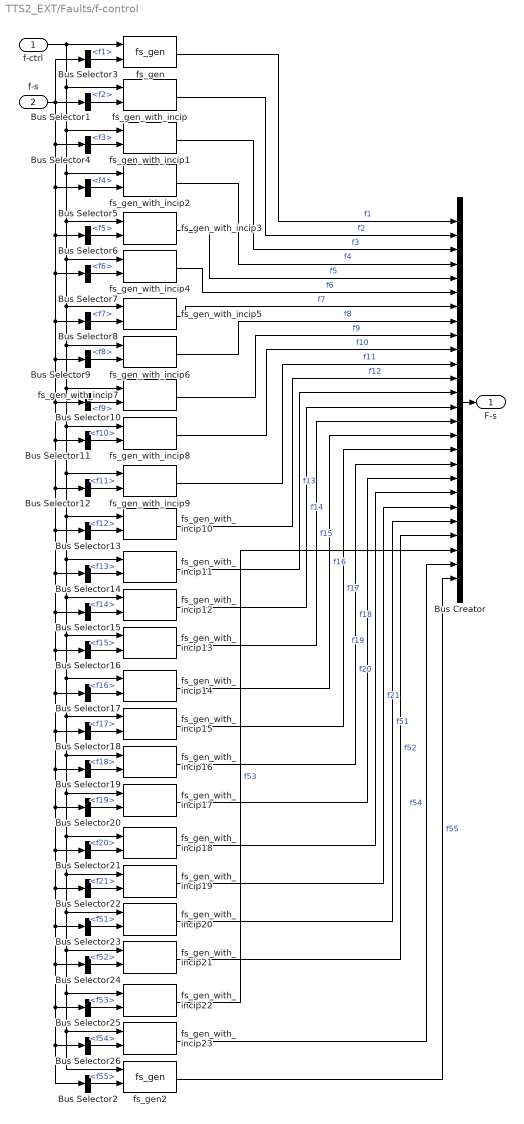
== system TTS2_EXT/Faults/f-control ==
  f-ctrl : Inport
  f-s : Inport  Port=2
  Bus Creator : BusCreator  Inputs=26
  Bus Selector1 : BusSelector  OutputSignals=f2
  Bus Selector10 : BusSelector  OutputSignals=f9
  Bus Selector11 : BusSelector  OutputSignals=f10
  Bus Selector12 : BusSelector  OutputSignals=f11
  Bus Selector13 : BusSelector  OutputSignals=f12
  Bus Selector14 : BusSelector  OutputSignals=f13
  Bus Selector15 : BusSelector  OutputSignals=f14
  Bus Selector16 : BusSelector  OutputSignals=f15
  Bus Selector17 : BusSelector  OutputSignals=f16
  Bus Selector18 : BusSelector  OutputSignals=f17
  Bus Selector19 : BusSelector  OutputSignals=f18
  Bus Selector2 : BusSelector  OutputSignals=f55
  Bus Selector20 : BusSelector  OutputSignals=f19
  Bus Selector21 : BusSelector  OutputSignals=f20
  Bus Selector22 : BusSelector  OutputSignals=f21
  Bus Selector23 : BusSelector  OutputSignals=f51
  Bus Selector24 : BusSelector  OutputSignals=f52
  Bus Selector25 : BusSelector  OutputSignals=f53
  Bus Selector26 : BusSelector  OutputSignals=f54
  Bus Selector3 : BusSelector  OutputSignals=f1
  Bus Selector4 : BusSelector  OutputSignals=f3
  Bus Selector5 : BusSelector  OutputSignals=f4
  Bus Selector6 : BusSelector  OutputSignals=f5
  Bus Selector7 : BusSelector  OutputSignals=f6
  Bus Selector8 : BusSelector  OutputSignals=f7
  Bus Selector9 : BusSelector  OutputSignals=f8
  fs_gen : lab310_library/fs_gen  p=p_f1  t=t_f1
  fs_gen2 : lab310_library/fs_gen  p=p_f55  t=t_f55
  fs_gen_with_incip : lab310_library/fs_gen_with_incip  p=p_f2  t=t_f2  st=st
  fs_gen_with_incip1 : lab310_library/fs_gen_with_incip  p=p_f3  t=t_f3  st=st
  fs_gen_with_incip10 : lab310_library/fs_gen_with_incip  p=p_f12  t=t_f12  st=st
  fs_gen_with_incip11 : lab310_library/fs_gen_with_incip  p=p_f13  t=t_f13  st=st
  fs_gen_with_incip12 : lab310_library/fs_gen_with_incip  p=p_f14  t=t_f14  st=st
  fs_gen_with_incip13 : lab310_library/fs_gen_with_incip  p=p_f15  t=t_f15  st=st
  fs_gen_with_incip14 : lab310_library/fs_gen_with_incip  p=p_f16  t=t_f16  st=st
  fs_gen_with_incip15 : lab310_library/fs_gen_with_incip  p=p_f17  t=t_f17  st=st
  fs_gen_with_incip16 : lab310_library/fs_gen_with_incip  p=p_f18  t=t_f18  st=st
  fs_gen_with_incip17 : lab310_library/fs_gen_with_incip  p=p_f19  t=t_f19  st=st
  fs_gen_with_incip18 : lab310_library/fs_gen_with_incip  p=p_f20  t=t_f20  st=st
  fs_gen_with_incip19 : lab310_library/fs_gen_with_incip  p=p_f21  t=t_f21  st=st
  fs_gen_with_incip2 : lab310_library/fs_gen_with_incip  p=p_f4  t=t_f4  st=st
  fs_gen_with_incip20 : lab310_library/fs_gen_with_incip  p=p_f51  t=t_f51  st=st
  fs_gen_with_incip21 : lab310_library/fs_gen_with_incip  p=p_f52  t=t_f52  st=st
  fs_gen_with_incip22 : lab310_library/fs_gen_with_incip  p=p_f53  t=t_f53  st=st
  fs_gen_with_incip23 : lab310_library/fs_gen_with_incip  p=p_f54  t=t_f54  st=st
  fs_gen_with_incip3 : lab310_library/fs_gen_with_incip  p=p_f5  t=t_f5  st=st
  fs_gen_with_incip4 : lab310_library/fs_gen_with_incip  p=p_f6  t=t_f6  st=st
  fs_gen_with_incip5 : lab310_library/fs_gen_with_incip  p=p_f7  t=t_f7  st=st
  fs_gen_with_incip6 : lab310_library/fs_gen_with_incip  p=p_f8  t=t_f8  st=st
  fs_gen_with_incip7 : lab310_library/fs_gen_with_incip  p=p_f9  t=t_f9  st=st
  fs_gen_with_incip8 : lab310_library/fs_gen_with_incip  p=p_f10  t=t_f10  st=st
  fs_gen_with_incip9 : lab310_library/fs_gen_with_incip  p=p_f11  t=t_f11  st=st
  F-s : Outport  VectorParamsAs1DForOutWhenUnconnected=off
  wires:
  Bus Creator/1 -> F-s/1
  fs_gen/1 -> Bus Creator/1  "f1"
  fs_gen_with_incip/1 -> Bus Creator/2  "f2"
  fs_gen_with_incip1/1 -> Bus Creator/3  "f3"
  fs_gen_with_incip2/1 -> Bus Creator/4  "f4"
  fs_gen_with_incip3/1 -> Bus Creator/5  "f5"
  fs_gen_with_incip4/1 -> Bus Creator/6  "f6"
  fs_gen_with_incip5/1 -> Bus Creator/7  "f7"
  fs_gen_with_incip6/1 -> Bus Creator/8  "f8"
  fs_gen_with_incip7/1 -> Bus Creator/9  "f9"
  fs_gen_with_incip8/1 -> Bus Creator/10  "f10"
  fs_gen_with_incip9/1 -> Bus Creator/11  "f11"
  f-s/1 -> Bus Selector1/1, Bus Selector3/1, Bus Selector4/1, Bus Selector5/1, Bus Selector6/1, Bus Selector7/1, Bus Selector8/1, Bus Selector9/1, Bus Selector10/1, Bus Selector11/1, Bus Selector12/1, Bus Selector13/1, Bus Selector14/1, Bus Selector15/1, Bus Selector16/1, Bus Selector17/1, Bus Selector18/1, Bus Selector19/1, Bus Selector20/1, Bus Selector21/1, Bus Selector22/1, Bus Selector23/1, Bus Selector24/1, Bus Selector25/1, Bus Selector26/1, Bus Selector2/1
  fs_gen_with_incip10/1 -> Bus Creator/12  "f12"
  fs_gen_with_incip11/1 -> Bus Creator/13  "f13"
  fs_gen_with_incip12/1 -> Bus Creator/14  "f14"
  fs_gen_with_incip13/1 -> Bus Creator/15  "f15"
  fs_gen_with_incip14/1 -> Bus Creator/16  "f16"
  fs_gen_with_incip15/1 -> Bus Creator/17  "f17"
  fs_gen_with_incip16/1 -> Bus Creator/18  "f18"
  fs_gen_with_incip17/1 -> Bus Creator/19  "f19"
  fs_gen_with_incip18/1 -> Bus Creator/20  "f20"
  fs_gen_with_incip19/1 -> Bus Creator/21  "f21"
  fs_gen_with_incip20/1 -> Bus Creator/22  "f51"
  fs_gen_with_incip21/1 -> Bus Creator/23  "f52"
  fs_gen_with_incip22/1 -> Bus Creator/24  "f53"
  fs_gen_with_incip23/1 -> Bus Creator/25  "f54"
  fs_gen2/1 -> Bus Creator/26  "f55"
  f-ctrl/1 -> fs_gen/1, fs_gen_with_incip/1, fs_gen_with_incip3/1, fs_gen_with_incip4/1, fs_gen2/1, fs_gen_with_incip23/1, fs_gen_with_incip22/1, fs_gen_with_incip21/1, fs_gen_with_incip20/1, fs_gen_with_incip19/1, fs_gen_with_incip18/1, fs_gen_with_incip17/1, fs_gen_with_incip16/1, fs_gen_with_incip15/1, fs_gen_with_incip14/1, fs_gen_with_incip13/1, fs_gen_with_incip12/1, fs_gen_with_incip11/1, fs_gen_with_incip10/1, fs_gen_with_incip9/1, fs_gen_with_incip8/1, fs_gen_with_incip7/1, fs_gen_with_incip6/1, fs_gen_with_incip5/1, fs_gen_with_incip2/1, fs_gen_with_incip1/1
  Bus Selector3/1 -> fs_gen/2  "<f1>"
  Bus Selector1/1 -> fs_gen_with_incip/2  "<f2>"
  Bus Selector2/1 -> fs_gen2/2  "<f55>"
  Bus Selector4/1 -> fs_gen_with_incip1/2  "<f3>"
  Bus Selector5/1 -> fs_gen_with_incip2/2  "<f4>"
  Bus Selector6/1 -> fs_gen_with_incip3/2  "<f5>"
  Bus Selector7/1 -> fs_gen_with_incip4/2  "<f6>"
  Bus Selector8/1 -> fs_gen_with_incip5/2  "<f7>"
  Bus Selector9/1 -> fs_gen_with_incip6/2  "<f8>"
  Bus Selector10/1 -> fs_gen_with_incip7/2  "<f9>"
  Bus Selector11/1 -> fs_gen_with_incip8/2  "<f10>"
  Bus Selector12/1 -> fs_gen_with_incip9/2  "<f11>"
  Bus Selector13/1 -> fs_gen_with_incip10/2  "<f12>"
  Bus Selector14/1 -> fs_gen_with_incip11/2  "<f13>"
  Bus Selector15/1 -> fs_gen_with_incip12/2  "<f14>"
  Bus Selector16/1 -> fs_gen_with_incip13/2  "<f15>"
  Bus Selector17/1 -> fs_gen_with_incip14/2  "<f16>"
  Bus Selector18/1 -> fs_gen_with_incip15/2  "<f17>"
  Bus Selector19/1 -> fs_gen_with_incip16/2  "<f18>"
  Bus Selector20/1 -> fs_gen_with_incip17/2  "<f19>"
  Bus Selector21/1 -> fs_gen_with_incip18/2  "<f20>"
  Bus Selector22/1 -> fs_gen_with_incip19/2  "<f21>"
  Bus Selector23/1 -> fs_gen_with_incip20/2  "<f51>"
  Bus Selector24/1 -> fs_gen_with_incip21/2  "<f52>"
  Bus Selector25/1 -> fs_gen_with_incip22/2  "<f53>"
  Bus Selector26/1 -> fs_gen_with_incip23/2  "<f54>"

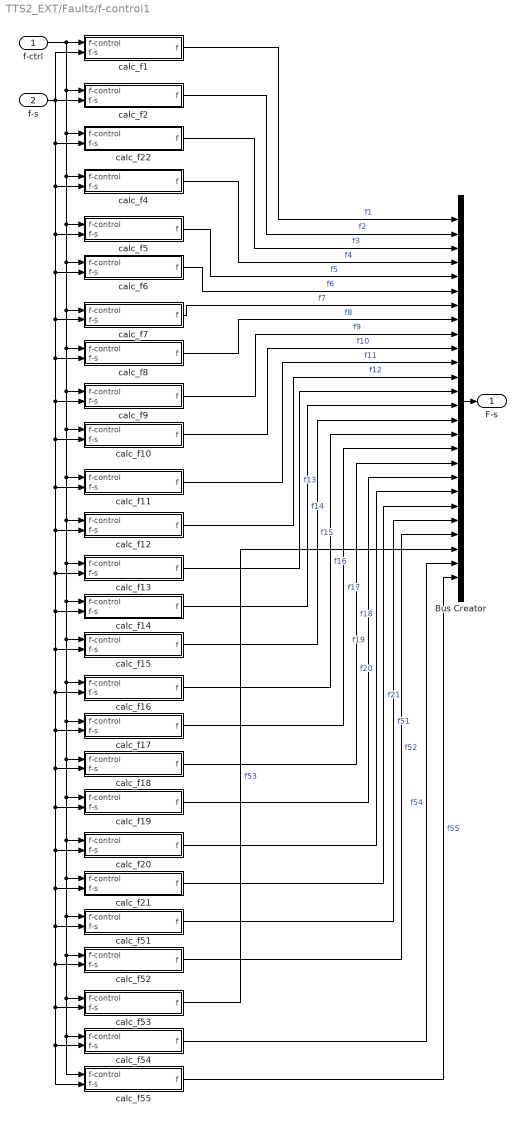
== system TTS2_EXT/Faults/f-control1 ==
  f-ctrl : Inport
  f-s : Inport  Port=2
  Bus Creator : BusCreator  Inputs=26
  calc_f1 : Subsystem  mask{p=p_f1, t=t_f1, st=st, amp=amp_f1, from=from_f1}
      mask prompts: p "Czy symulujemy?"; t "Czas startu"; st "Czas trwania"; amp "Amplituda (auto)"; from "Czas startu (auto)"
  calc_f10 : Subsystem  mask{p=p_f10, t=t_f10, st=st, amp=amp_f10, from=from_f10}
      mask prompts: p "Czy symulujemy?"; t "Czas startu"; st "Czas trwania"; amp "Amplituda (auto)"; from "Czas startu (auto)"
  calc_f11 : Subsystem  mask{p=p_f11, t=t_f11, st=st, amp=amp_f11, from=from_f11}
      mask prompts: p "Czy symulujemy?"; t "Czas startu"; st "Czas trwania"; amp "Amplituda (auto)"; from "Czas startu (auto)"
  calc_f12 : Subsystem  mask{p=p_f12, t=t_f12, st=st, amp=amp_f12, from=from_f12}
      mask prompts: p "Czy symulujemy?"; t "Czas startu"; st "Czas trwania"; amp "Amplituda (auto)"; from "Czas startu (auto)"
  calc_f13 : Subsystem  mask{p=p_f13, t=t_f13, st=st, amp=amp_f13, from=from_f13}
      mask prompts: p "Czy symulujemy?"; t "Czas startu"; st "Czas trwania"; amp "Amplituda (auto)"; from "Czas startu (auto)"
  calc_f14 : Subsystem  mask{p=p_f14, t=t_f14, st=st, amp=amp_f14, from=from_f14}
      mask prompts: p "Czy symulujemy?"; t "Czas startu"; st "Czas trwania"; amp "Amplituda (auto)"; from "Czas startu (auto)"
  calc_f15 : Subsystem  mask{p=p_f15, t=t_f15, st=st, amp=amp_f15, from=from_f15}
      mask prompts: p "Czy symulujemy?"; t "Czas startu"; st "Czas trwania"; amp "Amplituda (auto)"; from "Czas startu (auto)"
  calc_f16 : Subsystem  mask{p=p_f16, t=t_f16, st=st, amp=amp_f16, from=from_f16}
      mask prompts: p "Czy symulujemy?"; t "Czas startu"; st "Czas trwania"; amp "Amplituda (auto)"; from "Czas startu (auto)"
  calc_f17 : Subsystem  mask{p=p_f17, t=t_f17, st=st, amp=amp_f17, from=from_f17}
      mask prompts: p "Czy symulujemy?"; t "Czas startu"; st "Czas trwania"; amp "Amplituda (auto)"; from "Czas startu (auto)"
  calc_f18 : Subsystem  mask{p=p_f18, t=t_f18, st=st, amp=amp_f18, from=from_f18}
      mask prompts: p "Czy symulujemy?"; t "Czas startu"; st "Czas trwania"; amp "Amplituda (auto)"; from "Czas startu (auto)"
  calc_f19 : Subsystem  mask{p=p_f19, t=t_f19, st=st, amp=amp_f19, from=from_f19}
      mask prompts: p "Czy symulujemy?"; t "Czas startu"; st "Czas trwania"; amp "Amplituda (auto)"; from "Czas startu (auto)"
  calc_f2 : Subsystem  mask{p=p_f2, t=t_f2, st=st, amp=w_f2, from=from_f2}
      mask prompts: p "Czy symulujemy?"; t "Czas startu"; st "Czas trwania"; amp "Amplituda (auto)"; from "Czas startu (auto)"
  calc_f20 : Subsystem  mask{p=p_f20, t=t_f20, st=st, amp=amp_f20, from=from_f20}
      mask prompts: p "Czy symulujemy?"; t "Czas startu"; st "Czas trwania"; amp "Amplituda (auto)"; from "Czas startu (auto)"
  calc_f21 : Subsystem  mask{p=p_f21, t=t_f21, st=st, amp=amp_f21, from=from_f21}
      mask prompts: p "Czy symulujemy?"; t "Czas startu"; st "Czas trwania"; amp "Amplituda (auto)"; from "Czas startu (auto)"
  calc_f22 : Subsystem  mask{p=p_f3, t=t_f3, st=st, amp=amp_f3, from=from_f3}
      mask prompts: p "Czy symulujemy?"; t "Czas startu"; st "Czas trwania"; amp "Amplituda (auto)"; from "Czas startu (auto)"
  calc_f4 : Subsystem  mask{p=p_f4, t=t_f4, st=st, amp=amp_f4, from=from_f4}
      mask prompts: p "Czy symulujemy?"; t "Czas startu"; st "Czas trwania"; amp "Amplituda (auto)"; from "Czas startu (auto)"
  calc_f5 : Subsystem  mask{p=p_f5, t=t_f5, st=st, amp=amp_f5, from=from_f5}
      mask prompts: p "Czy symulujemy?"; t "Czas startu"; st "Czas trwania"; amp "Amplituda (auto)"; from "Czas startu (auto)"
  calc_f51 : Subsystem  mask{p=p_f51, t=t_f51, st=st, amp=amp_f51, from=from_f51}
      mask prompts: p "Czy symulujemy?"; t "Czas startu"; st "Czas trwania"; amp "Amplituda (auto)"; from "Czas startu (auto)"
  calc_f52 : Subsystem  mask{p=p_f52, t=t_f52, st=st, amp=amp_f52, from=from_f52}
      mask prompts: p "Czy symulujemy?"; t "Czas startu"; st "Czas trwania"; amp "Amplituda (auto)"; from "Czas startu (auto)"
  calc_f53 : Subsystem  mask{p=p_f53, t=t_f53, st=st, amp=amp_f53, from=from_f53}
      mask prompts: p "Czy symulujemy?"; t "Czas startu"; st "Czas trwania"; amp "Amplituda (auto)"; from "Czas startu (auto)"
  calc_f54 : Subsystem  mask{p=p_f54, t=t_f54, st=st, amp=amp_f54, from=from_f54}
      mask prompts: p "Czy symulujemy?"; t "Czas startu"; st "Czas trwania"; amp "Amplituda (auto)"; from "Czas startu (auto)"
  calc_f55 : Subsystem  mask{p=p_f55, t=t_f55, st=st, amp=amp_f55, from=from_f55}
      mask prompts: p "Czy symulujemy?"; t "Czas startu"; st "Czas trwania"; amp "Amplituda (auto)"; from "Czas startu (auto)"
  calc_f6 : Subsystem  mask{p=p_f6, t=t_f6, st=st, amp=amp_f6, from=from_f6}
      mask prompts: p "Czy symulujemy?"; t "Czas startu"; st "Czas trwania"; amp "Amplituda (auto)"; from "Czas startu (auto)"
  calc_f7 : Subsystem  mask{p=p_f7, t=t_f7, st=st, amp=amp_f7, from=from_f7}
      mask prompts: p "Czy symulujemy?"; t "Czas startu"; st "Czas trwania"; amp "Amplituda (auto)"; from "Czas startu (auto)"
  calc_f8 : Subsystem  mask{p=p_f8, t=t_f8, st=st, amp=amp_f8, from=from_f8}
      mask prompts: p "Czy symulujemy?"; t "Czas startu"; st "Czas trwania"; amp "Amplituda (auto)"; from "Czas startu (auto)"
  calc_f9 : Subsystem  mask{p=p_f9, t=t_f9, st=st, amp=amp_f9, from=from_f9}
      mask prompts: p "Czy symulujemy?"; t "Czas startu"; st "Czas trwania"; amp "Amplituda (auto)"; from "Czas startu (auto)"
  F-s : Outport  VectorParamsAs1DForOutWhenUnconnected=off
  wires:
  Bus Creator/1 -> F-s/1
  calc_f1/1(f) -> Bus Creator/1  "f1"
  calc_f2/1(f) -> Bus Creator/2  "f2"
  calc_f22/1(f) -> Bus Creator/3  "f3"
  calc_f4/1(f) -> Bus Creator/4  "f4"
  calc_f5/1(f) -> Bus Creator/5  "f5"
  calc_f6/1(f) -> Bus Creator/6  "f6"
  calc_f7/1(f) -> Bus Creator/7  "f7"
  calc_f8/1(f) -> Bus Creator/8  "f8"
  calc_f9/1(f) -> Bus Creator/9  "f9"
  calc_f10/1(f) -> Bus Creator/10  "f10"
  calc_f11/1(f) -> Bus Creator/11  "f11"
  f-s/1 -> calc_f1/2(f-s), calc_f2/2(f-s), calc_f22/2(f-s), calc_f4/2(f-s), calc_f5/2(f-s), calc_f6/2(f-s), calc_f7/2(f-s), calc_f8/2(f-s), calc_f9/2(f-s), calc_f10/2(f-s), calc_f11/2(f-s), calc_f12/2(f-s), calc_f13/2(f-s), calc_f14/2(f-s), calc_f15/2(f-s), calc_f16/2(f-s), calc_f17/2(f-s), calc_f18/2(f-s), calc_f19/2(f-s), calc_f20/2(f-s), calc_f21/2(f-s), calc_f51/2(f-s), calc_f52/2(f-s), calc_f53/2(f-s), calc_f55/2(f-s), calc_f54/2(f-s)
  calc_f12/1(f) -> Bus Creator/12  "f12"
  calc_f13/1(f) -> Bus Creator/13  "f13"
  calc_f14/1(f) -> Bus Creator/14  "f14"
  calc_f15/1(f) -> Bus Creator/15  "f15"
  f-ctrl/1 -> calc_f1/1(f-control), calc_f2/1(f-control), calc_f22/1(f-control), calc_f4/1(f-control), calc_f5/1(f-control), calc_f6/1(f-control), calc_f7/1(f-control), calc_f8/1(f-control), calc_f9/1(f-control), calc_f10/1(f-control), calc_f11/1(f-control), calc_f12/1(f-control), calc_f13/1(f-control), calc_f14/1(f-control), calc_f15/1(f-control), calc_f16/1(f-control), calc_f17/1(f-control), calc_f18/1(f-control), calc_f19/1(f-control), calc_f20/1(f-control), calc_f21/1(f-control), calc_f51/1(f-control), calc_f52/1(f-control), calc_f53/1(f-control), calc_f55/1(f-control), calc_f54/1(f-control)
  calc_f16/1(f) -> Bus Creator/16  "f16"
  calc_f17/1(f) -> Bus Creator/17  "f17"
  calc_f18/1(f) -> Bus Creator/18  "f18"
  calc_f19/1(f) -> Bus Creator/19  "f19"
  calc_f20/1(f) -> Bus Creator/20  "f20"
  calc_f21/1(f) -> Bus Creator/21  "f21"
  calc_f51/1(f) -> Bus Creator/22  "f51"
  calc_f52/1(f) -> Bus Creator/23  "f52"
  calc_f53/1(f) -> Bus Creator/24  "f53"
  calc_f54/1(f) -> Bus Creator/25  "f54"
  calc_f55/1(f) -> Bus Creator/26  "f55"

== system TTS2_EXT/Monitoring & Analysis/Export data ==
  SP : Inport
  CV : Inport  Port=2
  PV : Inport  Port=3
  data : Inport  Port=4
  CVG1 : Inport  Port=5
  CVG2 : Inport  Port=6
  conf : Inport  Port=7
  Mux : Mux  Inputs=7
  To Workspace : ToWorkspace  VariableName=simout  SampleTime=-1
  wires:
  Mux/1 -> To Workspace/1
  CV/1 -> Mux/2
  SP/1 -> Mux/1
  PV/1 -> Mux/3
  data/1 -> Mux/4
  CVG1/1 -> Mux/5
  CVG2/1 -> Mux/6
  conf/1 -> Mux/7

== system TTS2_EXT/Monitoring & Analysis/Scopes ==
  e : Inport
  SP : Inport  Port=2
  CV : Inport  Port=3
  data : Inport  Port=4
  Bus Selector : BusSelector  OutputSignals=P1,G1,F1,F2,L11,L21,L31,L12,L22,L32
  CV,G1' : Scope  NumInputPorts=2
  Demux : Demux  Outputs=3
  F1',F2' : Scope  NumInputPorts=2
  "L11',L21',L32' " : Scope  NumInputPorts=3
  "P1' " : Scope
  SP,PV : Scope  NumInputPorts=2
  Scope : Scope  NumInputPorts=3
  "ep,ei,ed " : Scope  NumInputPorts=3
  wires:
  Bus Selector/3 -> F1',F2'/1  "<F1>"
  Bus Selector/9 -> Scope/2  "<L22>"
  Bus Selector/8 -> Scope/1  "<L12>"
  Demux/3 -> "ep,ei,ed "/3
  Demux/2 -> "ep,ei,ed "/2
  Bus Selector/10 -> Scope/3  "<L32>"
  Bus Selector/1 -> "P1' "/1  "<P1>"
  Demux/1 -> "ep,ei,ed "/1
  SP/1 -> SP,PV/1
  Bus Selector/4 -> F1',F2'/2  "<F2>"
  Bus Selector/6 -> "L11',L21',L32' "/2  "<L21>"
  Bus Selector/7 -> "L11',L21',L32' "/3, SP,PV/2  "<L31>"
  Bus Selector/5 -> "L11',L21',L32' "/1  "<L11>"
  e/1 -> Demux/1
  CV/1 -> CV,G1'/1
  Bus Selector/2 -> CV,G1'/2  "<G1>"
  data/1 -> Bus Selector/1
